simulink model "PassengerCar"  (R2019b)
settings: Solver=ode1  StartTime=0  StopTime=25  FixedStep=1.0000000000000000e-003  RelTol=1e-3
InitFcn:
  | sampleTime = str2double(get_param(bdroot, 'FixedStep'));
undefined symbols (not defined in the file or in its folder): AccPedalPos, BrakePedalPos, BrakeSwitch, DiscIntNeverNeededParam, DYNA4, EngSpd, IgnitionSwitch, InitialGear, InitialSpeed, IntendedEngTrq, LeftIndicator, MainBrakePress, MaxGear, MDL, MinGear, RefAcc, RefLane, RefLatPos, RefPath, RefPathCurv, RefSpd, RefSpdPreview, RefSpdRetrospect, RightIndicator, SteeringWheelAng, SteeringWheelTrq, UserDefinedRefValue, vm_const
libraries: UtilitiesLibrary x31, simulink x18, WheelSystemModules x13, LongitudinalControllerModules x13, LateralControllerModules x7, AnimationBusselectorModules x5, EnvironmentModules x5, BasicEngineControlModules x5, MiscellaneousControlModules x5, Animation3Modules x4, AuxiliariesModules x4, TireModules x4
(part 18 of 39)

== system PassengerCar/Vehicle/Drivetrain/DrivetrainControlUnit/InputFromDrivetrainPhysics ==
  fromDrivetrainPhysics : Inport
  TDBusSelector : BusSelector  OutputSignals=Transmission.Type[-],EngSpd[rad/s],Transmission.InSpd[rad/s],Transmission.OutSpd[rad/s],Transmission.NumFwdGears[-]
  __TDD__EngSpd[rad/s] : Demux  Outputs=[1]
  __TDD__InSpd[rad/s] : Demux  Outputs=[1]
  __TDD__NumFwdGears[-] : Demux  Outputs=[1]
  __TDD__OutSpd[rad/s] : Demux  Outputs=[1]
  __TDD__Type[-] : Demux  Outputs=1
  Type[-]___UNIQUE_1 : Outport  Description=|  VectorParamsAs1DForOutWhenUnconnected=off
      | <name>Transmission.Type[-]</name>
      | <comment></comment>
  EngSpd[rad/s] : Outport  Description=|  Port=2  PortDimensions=[1]  VectorParamsAs1DForOutWhenUnconnected=off
      | <name>EngSpd[rad/s]</name>
      | <comment>Engine speed</comment>
  InSpd[rad/s]___UNIQUE_1 : Outport  Description=|  Port=3  PortDimensions=[1]  VectorParamsAs1DForOutWhenUnconnected=off
      | <name>Transmission.InSpd[rad/s]</name>
      | <comment>Transmission input speed</comment>
  OutSpd[rad/s]___UNIQUE_1 : Outport  Description=|  Port=4  PortDimensions=[1]  VectorParamsAs1DForOutWhenUnconnected=off
      | <name>Transmission.OutSpd[rad/s]</name>
      | <comment>Transmission output speed</comment>
  NumFwdGears[-]___UNIQUE_1 : Outport  Description=|  Port=5  PortDimensions=[1]  VectorParamsAs1DForOutWhenUnconnected=off
      | <name>Transmission.NumFwdGears[-]</name>
      | <comment>Number of forward gears</comment>
  wires:
  __TDD__NumFwdGears[-]/1 -> NumFwdGears[-]___UNIQUE_1/1  "NumFwdGears[-]"
  __TDD__OutSpd[rad/s]/1 -> OutSpd[rad/s]___UNIQUE_1/1  "OutSpd[rad/s]"
  __TDD__InSpd[rad/s]/1 -> InSpd[rad/s]___UNIQUE_1/1  "InSpd[rad/s]"
  __TDD__EngSpd[rad/s]/1 -> EngSpd[rad/s]/1  "EngSpd[rad/s]"
  __TDD__Type[-]/1 -> Type[-]___UNIQUE_1/1  "Type[-]"
  TDBusSelector/5 -> __TDD__NumFwdGears[-]/1  "<NumFwdGears[-]>"
  TDBusSelector/4 -> __TDD__OutSpd[rad/s]/1  "<OutSpd[rad/s]>"
  TDBusSelector/3 -> __TDD__InSpd[rad/s]/1  "<InSpd[rad/s]>"
  TDBusSelector/2 -> __TDD__EngSpd[rad/s]/1  "<EngSpd[rad/s]>"
  TDBusSelector/1 -> __TDD__Type[-]/1  "<Type[-]>"
  fromDrivetrainPhysics/1 -> TDBusSelector/1

== system PassengerCar/Vehicle/Drivetrain/DrivetrainControlUnit/TransmissionControlUnit ==
  AccPedalPos[0_1] : Inport  Description=Accelerator pedal position
  EngSpd[rad/s] : Inport  Description=Engine speed  Port=2
  TransmissionInSpd[rad/s] : Inport  Description=Transmission input speed  Port=3
  TransmissionOutSpd[rad/s] : Inport  Description=Transmission output speed  Port=4
  NumFwdGears[-] : Inport  Description=Number of forward gears  Port=5
  InitialGear[-4;20] : Inport  Description=Accelerator pedal position  Port=6
  MaxGear[-4;20] : Inport  Description=Maximum gear  Port=7
  MinGear[-4;20] : Inport  Description=Minimum gear  Port=8
  ShiftingProgramSelection[-] : Inport  Description=Shifting program selection  Port=9
  KickdownSwitch[0;1] : Inport  Description=Kick-down switch  Port=10
  Enable : EnablePort  StatesWhenEnabling=reset
  TransmissionControlUnit : TransmissionControlModules/TransmissionControlUnit  DATA_NODE=MDL.Vehicle.Drivetrain.DrivetrainControlUnit.TransmissionControlUnit  GearChangeMinTime=MDL.Vehicle.Drivetrain.DrivetrainControlUnit.TransmissionControlUnit.GearChangeMinTime  GearChangeDelay=MDL.Vehicle.Drivetrain.DrivetrainControlUnit.TransmissionControlUnit.GearChangeDelay  EngSpdFilterTimeConst=MDL.Vehicle.Drivetrain.DrivetrainControlUnit.TransmissionControlUnit.EngSpdFilterTimeConst  LockUpClutchOpenTime=MDL.Vehicle.Drivetrain.DrivetrainControlUnit.TransmissionControlUnit.LockUpClutch.OpenTime  LockUpClutchCloseTime=MDL.Vehicle.Drivetrain.DrivetrainControlUnit.TransmissionControlUnit.LockUpClutch.CloseTime  ThresKickdownOpenControlled=MDL.Vehicle.Drivetrain.DrivetrainControlUnit.TransmissionControlUnit.LockUpClutch.KickDownMode.OpenToControlledSpdCurve  ThresKickdownControlledOpen=MDL.Vehicle.Drivetrain.DrivetrainControlUnit.TransmissionControlUnit.LockUpClutch.KickDownMode.ControlledToOpenSpdCurve  ThresKickdownClosedControlled=MDL.Vehicle.Drivetrain.DrivetrainControlUnit.TransmissionControlUnit.LockUpClutch.KickDownMode.ClosedToControlledSpdCurve  ThresKickdownControlledClosed=MDL.Vehicle.Drivetrain.DrivetrainControlUnit.TransmissionControlUnit.LockUpClutch.KickDownMode.ControlledToClosedSpdCurve  ThresOpenControlled=MDL.Vehicle.Drivetrain.DrivetrainControlUnit.TransmissionControlUnit.LockUpClutch.RegularMode.OpenToControlledSpdMap3D  ThresControlledOpen=MDL.Vehicle.Drivetrain.DrivetrainControlUnit.TransmissionControlUnit.LockUpClutch.RegularMode.ControlledToOpenSpdMap3D  ThresClosedControlled=MDL.Vehicle.Drivetrain.DrivetrainControlUnit.TransmissionControlUnit.LockUpClutch.RegularMode.ClosedToControlledSpdMap3D  ThresControlledClosed=MDL.Vehicle.Drivetrain.DrivetrainControlUnit.TransmissionControlUnit.LockUpClutch.RegularMode.ControlledToClosedSpdMap3D  OpenClutchDelay=MDL.Vehicle.Drivetrain.DrivetrainControlUnit.TransmissionControlUnit.ManualClutch.OpenClutchDelay  ClutchPedalCorrectFac=MDL.Vehicle.Drivetrain.DrivetrainControlUnit.TransmissionControlUnit.ManualClutch.ClutchPedalCorrectFacCurve  ClutchOpenTime=MDL.Vehicle.Drivetrain.DrivetrainControlUnit.TransmissionControlUnit.ManualClutch.OpenTime  OpenClutchDuration=MDL.Vehicle.Drivetrain.DrivetrainControlUnit.TransmissionControlUnit.ManualClutch.OpenClutchDuration  ClutchCloseTime=MDL.Vehicle.Drivetrain.DrivetrainControlUnit.TransmissionControlUnit.ManualClutch.CloseTime  LowerGearLimit=MDL.Vehicle.Drivetrain.DrivetrainControlUnit.TransmissionControlUnit.ShiftingProgram.DirectShifting.LowerGearLimit  TransmissionOutSpdThres=MDL.Vehicle.Drivetrain.DrivetrainControlUnit.TransmissionControlUnit.ShiftingProgram.DirectShifting.Spd  KickdownShiftUp=MDL.Vehicle.Drivetrain.DrivetrainControlUnit.TransmissionControlUnit.ShiftingProgram.KickDownMode.UpshiftSpdCurve  KickdownShiftDown=MDL.Vehicle.Drivetrain.DrivetrainControlUnit.TransmissionControlUnit.ShiftingProgram.KickDownMode.DownshiftSpdCurve  ShiftUp=MDL.Vehicle.Drivetrain.DrivetrainControlUnit.TransmissionControlUnit.ShiftingProgram.RegularMode.UpshiftSpdMap3D  ShiftDown=MDL.Vehicle.Drivetrain.DrivetrainControlUnit.TransmissionControlUnit.ShiftingProgram.RegularMode.DownshiftSpdMap3D  SlipCtrlClutchSlip=MDL.Vehicle.Drivetrain.DrivetrainControlUnit.TransmissionControlUnit.SlipController.ClutchIntendedSlipMap3D  SlipCtrlProportionalGain=MDL.Vehicle.Drivetrain.DrivetrainControlUnit.TransmissionControlUnit.SlipController.ProportionalGain  SlipCtrlIntegralGain=MDL.Vehicle.Drivetrain.DrivetrainControlUnit.TransmissionControlUnit.SlipController.IntegralGain  SlipCtrlTimeConst=MDL.Vehicle.Drivetrain.DrivetrainControlUnit.TransmissionControlUnit.SlipController.TimeConst  TractionCtrlIntTrq=MDL.Vehicle.Drivetrain.DrivetrainControlUnit.TransmissionControlUnit.TractionController.RefEngTrq  ASREndClutchPos=MDL.Vehicle.Drivetrain.DrivetrainControlUnit.TransmissionControlUnit.TractionController.ASREndClutchPos
  Gear[-4;20] : Outport  Description=Gear  OutputWhenDisabled=reset  InitialOutput=0  VectorParamsAs1DForOutWhenUnconnected=off
  LockUpClutchPos[0_1] : Outport  Description=Lock-up clutch position  Port=2  OutputWhenDisabled=reset  InitialOutput=0  VectorParamsAs1DForOutWhenUnconnected=off
  AutomatedManualClutchPos[0_1] : Outport  Description=Clutch position for manual shifting  Port=3  OutputWhenDisabled=reset  InitialOutput=0  VectorParamsAs1DForOutWhenUnconnected=off
  GearTarget[-4;20] : Outport  Description=ASR torque  Port=4  OutputWhenDisabled=reset  InitialOutput=0  VectorParamsAs1DForOutWhenUnconnected=off
  ASRRequestSwitch[0;2] : Outport  Description=Switch indicating if no ASR (0), slow ASR (1), or fast ASR (2) is requested  Port=5  OutputWhenDisabled=reset  InitialOutput=0  VectorParamsAs1DForOutWhenUnconnected=off
  ASRTrq[Nm] : Outport  Description=ASR torque  Port=6  OutputWhenDisabled=reset  InitialOutput=0  VectorParamsAs1DForOutWhenUnconnected=off
  wires:
  InitialGear[-4;20]/1 -> TransmissionControlUnit/6
  NumFwdGears[-]/1 -> TransmissionControlUnit/5
  TransmissionOutSpd[rad/s]/1 -> TransmissionControlUnit/4
  EngSpd[rad/s]/1 -> TransmissionControlUnit/2
  AccPedalPos[0_1]/1 -> TransmissionControlUnit/1
  TransmissionInSpd[rad/s]/1 -> TransmissionControlUnit/3
  KickdownSwitch[0;1]/1 -> TransmissionControlUnit/10
  TransmissionControlUnit/6 -> GearTarget[-4;20]/1
  ShiftingProgramSelection[-]/1 -> TransmissionControlUnit/9
  MinGear[-4;20]/1 -> TransmissionControlUnit/8
  MaxGear[-4;20]/1 -> TransmissionControlUnit/7
  TransmissionControlUnit/1 -> Gear[-4;20]/1
  TransmissionControlUnit/2 -> LockUpClutchPos[0_1]/1
  TransmissionControlUnit/3 -> AutomatedManualClutchPos[0_1]/1
  TransmissionControlUnit/4 -> ASRRequestSwitch[0;2]/1
  TransmissionControlUnit/5 -> ASRTrq[Nm]/1

== system PassengerCar/Vehicle/Drivetrain/DrivetrainPhysics/DrivetrainPhysicsInputs ==
  fromEngine : Inport
  fromWheelSystem : Inport  Port=2
  fromCTRL : Inport  Port=3
  fromDrivetrainControlUnit : Inport  Port=4
  fromAuxiliaries : Inport  Port=5
  Add : Sum
  Add1 : Sum
  Add2 : Sum  Inputs=+-
  Bus to Vector : BusToVector
  InputFromAuxiliaries : Subsystem  Tag=TESIS DYNAware Interface Block  mask{NeedsUpdate=off, SignalInfo=|}
      mask SignalInfo=|
      | {
      |   "Version": "4.6",
      |   "MuxedOutputBusName": "output",
      |   "MuxedInputBusName": "fromAuxiliaries",
      |   "MuxedInputSelected": true,
      |   "MuxedOutputSelected": false,
      |   "SignalData": [
      |     {
      |       "initialValue": "0.0",
      |       "name": "StarterInrt[kgm**2]",
      |       "comment": "",
      |       "minString": "",
      |       "maxString": "",
      |       "width": 1,
      |       "dataType": 0,
      |       "signalType": 0,
      |       "createSignal": false,
      |       "outputName": "StarterInrt[kgm**2]",
      |       "generateSignalAccessBlock": false,
      |       "accessId": "$(parentId).$(blockName).$(outputName)"
      |     },
      |     {
      |       "initialValue": "0.0",
      |       "name": "StarterTrq[Nm]",
      |       "comment": "",
      |       "minString": "",
      |       "maxString": "",
      |       "width": 1,
      |       "dataType": 0,
      |       "signalType": 0,
      |       "createSignal": false,
      |       "outputName": "StarterTrq[Nm]",
      |       "generateSignalAccessBlock": false,
      |       "accessId": "$(parentId).$(blockName).$(outputName)"
      |     }
      |   ]
      | }
      mask prompts: NeedsUpdate "Specify, if subsystem content needs to be updated"; SignalInfo "Signal Info (json)"
      mask help: DYNA4 Interface Block Version 4.6
      mask init:
      | blockName = get_param(gcbh, 'Name');
      | parentId = DYNA4.ModelHandling.AccessID.getFromHierarchy(gcbh);
      | TD.InterfaceBlock.ModelCallbacks.GenerateContent(gcb);
      settings: DeleteFcn=TD.InterfaceBlock.ModelCallbacks.CloseGUI( gcbh );  NameChangeFcn=TD.InterfaceBlock.ModelCallbacks.BlockRenamedHandler(gcbh);  OpenFcn=TD.InterfaceBlock.ModelCallbacks.OpenGUI( gcbh );  CloseFcn=TD.InterfaceBlock.ModelCallbacks.CloseGUI( gcbh );
      mask Display:
      | image('InterfaceBlock.png','center');
      | port_label('input',1, 'fromAuxiliaries');
      | port_label('output',1, 'StarterInrt[kgm**2]');
      | port_label('output',2, 'StarterTrq[Nm]');
  InputFromCTRL : Subsystem  Tag=TESIS DYNAware Interface Block  mask{NeedsUpdate=off, SignalInfo=|}
      mask SignalInfo=|
      | {
      |   "Version": "4.6",
      |   "MuxedOutputBusName": "output",
      |   "MuxedInputBusName": "fromCTRL",
      |   "MuxedInputSelected": true,
      |   "MuxedOutputSelected": false,
      |   "SignalData": [
      |     {
      |       "initialValue": "0.0",
      |       "name": "CTRL.LongitudinalControl.InitialEngineSpeed[rad/s]",
      |       "comment": "",
      |       "minString": "",
      |       "maxString": "",
      |       "width": 1,
      |       "dataType": 0,
      |       "signalType": 0,
      |       "createSignal": false,
      |       "outputName": "InitialEngineSpeed[rad/s]",
      |       "generateSignalAccessBlock": false,
      |       "accessId": "$(parentId).$(blockName).$(outputName)"
      |     },
      |     {
      |       "initialValue": "0.0",
      |       "name": "CTRL.LongitudinalControl.InitialGear[-4;20]",
      |       "comment": "",
      |       "minString": "",
      |       "maxString": "",
      |       "width": 1,
      |       "dataType": 0,
      |       "signalType": 0,
      |       "createSignal": false,
      |       "outputName": "InitialGear[-4;20]",
      |       "generateSignalAccessBlock": false,
      |       "accessId": "$(parentId).$(blockName).$(outputName)"
      |     },
      |     {
      |       "initialValue": "0.0",
      |       "name": "CTRL.LongitudinalControl.ClutchPos[0_1]",
      |       "comment": "",
      |       "minString": "",
      |       "maxString": "",
      |       "width": 1,
      |       "dataType": 0,
      |       "signalType": 0,
      |       "createSignal": false,
      |       "outputName": "ClutchPos[0_1]",
      |       "generateSignalAccessBlock": false,
      |       "accessId": "$(parentId).$(blockName).$(outputName)"
      |     },
      |     {
      |       "initialValue": "0.0",
      |       "name": "CTRL.LongitudinalControl.ManualGear[-4;20]",
      |       "comment": "",
      |       "minString": "",
      |       "maxString": "",
      |       "width": 1,
      |       "dataType": 0,
      |       "signalType": 0,
      |       "createSignal": false,
      |       "outputName": "ManualGear[-4;20]",
      |       "generateSignalAccessBlock": false,
      |       "accessId": "$(parentId).$(blockName).$(outputName)"
      |     },
      |     {
      |       "initialValue": "0.0",
      |       "name": "CTRL.LongitudinalControl.TransferCaseLock[0;1]",
      |       "comment": "",
      |       "minString": "",
      |       "maxString": "",
      |       "width": 1,
      |       "dataType": 0,
      |       "signalType": 0,
      |       "createSignal": false,
      |       "outputName": "TransferCaseLock[0;1]",
      |       "generateSignalAccessBlock": false,
      |       "accessId": "$(parentId).$(blockName).$(outputName)"
      |     },
      |     {
      |       "initialValue": "0.0",
      |       "name": "CTRL.LongitudinalControl.FrontDifferentialLock[0;1]",
      |       "comment": "",
      |       "minString": "",
      |       "maxString": "",
      |       "width": 1,
      |       "dataType": 0,
      |       "signalType": 0,
      |       "createSignal": false,
      |       "outputName": "FrontDifferentialLock[0;1]",
      |       "generateSignalAccessBlock": false,
      |       "accessId": "$(parentId).$(blockName).$(outputName)"
      |     },
      |     {
      |       "initialValue": "0.0",
      |       "name": "CTRL.LongitudinalControl.RearDifferentialLock[0;1]",
      |       "comment": "",
      |       "minString": "",
      |       "maxString": "",
      |       "width": 1,
      |       "dataType": 0,
      |       "signalType": 0,
      |       "createSignal": false,
      |       "outputName": "RearDifferentialLock[0;1]",
      |       "generateSignalAccessBlock": false,
      |       "accessId": "$(parentId).$(blockName).$(outputName)"
      |     },
      |     {
      |       "initialValue": "0.0",
      |       "name": "CTRL.LongitudinalControl.Rear2DifferentialLock[0;1]",
      |       "comment": "",
      |       "minString": "",
      |       "maxString": "",
      |       "width": 1,
      |       "dataType": 0,
      |       "signalType": 0,
      |       "createSignal": false,
      |       "outputName": "Rear2DifferentialLock[0;1]",
      |       "generateSignalAccessBlock": false,
      |       "accessId": "$(parentId).$(blockName).$(outputName)"
      |     },
      |     {
      |       "initialValue": "0.0",
      |       "name": "CTRL.LongitudinalControl.Rear3DifferentialLock[0;1]",
      |       "comment": "",
      |       "minString": "",
      |       "maxString": "",
      |       "width": 1,
      |       "dataType": 0,
      |       "signalType": 0,
      |       "createSignal": false,
      |       "outputName": "Rear3DifferentialLock[0;1]",
      |       "generateSignalAccessBlock": false,
      |       "accessId": "$(parentId).$(blockName).$(outputName)"
      |     },
      |     {
      |       "initialValue": "0.0",
      |       "name": "CTRL.TemperatureControl.TransmissionTemp[K]",
      |       "comment": "",
      |       "minString": "",
      |       "maxString": "",
      |       "width": 1,
      |       "dataType": 0,
      |       "signalType": 0,
      |       "createSignal": false,
      |       "outputName": "TransmissionTemp[K]",
      |       "generateSignalAccessBlock": false,
      |       "accessId": "$(parentId).$(blockName).$(outputName)"
      |     },
      |     {
      |       "initialValue": "0.0",
      |       "name": "CTRL.TemperatureControl.TransferCaseTemp[K]",
      |       "comment": "",
      |       "minString": "",
      |       "maxString": "",
      |       "width": 1,
      |       "dataType": 0,
      |       "signalType": 0,
      |       "createSignal": false,
      |       "outputName": "TransferCaseTemp[K]",
      |       "generateSignalAccessBlock": false,
      |       "accessId": "$(parentId).$(blockName).$(outputName)"
      |     },
      |     {
      |       "initialValue": "0.0",
      |       "name": "CTRL.TemperatureControl.FrontDifferentialTemp[K]",
      |       "comment": "",
      |       "minString": "",
      |       "maxString": "",
      |       "width": 1,
      |       "dataType": 0,
      |       "signalType": 0,
      |       "createSignal": false,
      |       "outputName": "FrontDifferentialTemp[K]",
      |       "generateSignalAccessBlock": false,
      |       "accessId": "$(parentId).$(blockName).$(outputName)"
      |     },
      |     {
      |       "initialValue": "0.0",
      |       "name": "CTRL.TemperatureControl.RearDifferentialTemp[K]",
      |       "comment": "",
      |       "minString": "",
      |       "maxString": "",
      |       "width": 1,
      |       "dataType": 0,
      |       "signalType": 0,
      |       "createSignal": false,
      |       "outputName": "RearDifferentialTemp[K]",
      |       "generateSignalAccessBlock": false,
      |       "accessId": "$(parentId).$(blockName).$(outputName)"
      |     },
      |     {
      |       "initialValue": "0.0",
      |       "name": "CTRL.TemperatureControl.Rear2DifferentialTemp[K]",
      |       "comment": "",
      |       "minString": "",
      |       "maxString": "",
      |       "width": 1,
      |       "dataType": 0,
      |       "signalType": 0,
      |       "createSignal": false,
      |       "outputName": "Rear2DifferentialTemp[K]",
      |       "generateSignalAccessBlock": false,
      |       "accessId": "$(parentId).$(blockName).$(outputName)"
      |     },
      |     {
      |       "initialValue": "0.0",
      |       "name": "CTRL.TemperatureControl.Rear3DifferentialTemp[K]",
      |       "comment": "",
      |       "minString": "",
      |       "maxString": "",
      |       "width": 1,
      |       "dataType": 0,
      |       "signalType": 0,
      |       "createSignal": false,
      |       "outputName": "Rear3DifferentialTemp[K]",
      |       "generateSignalAccessBlock": false,
      |       "accessId": "$(parentId).$(blockName).$(outputName)"
      |     }
      |   ]
      | }
      mask prompts: NeedsUpdate "Specify, if subsystem content needs to be updated"; SignalInfo "Signal Info (json)"
      mask help: DYNA4 Interface Block Version 4.6
      mask init:
      | blockName = get_param(gcbh, 'Name');
      | parentId = DYNA4.ModelHandling.AccessID.getFromHierarchy(gcbh);
      | TD.InterfaceBlock.ModelCallbacks.GenerateContent(gcb);
      settings: DeleteFcn=TD.InterfaceBlock.ModelCallbacks.CloseGUI( gcbh );  NameChangeFcn=TD.InterfaceBlock.ModelCallbacks.BlockRenamedHandler(gcbh);  OpenFcn=TD.InterfaceBlock.ModelCallbacks.OpenGUI( gcbh );  CloseFcn=TD.InterfaceBlock.ModelCallbacks.CloseGUI( gcbh );
      mask Display:
      | image('InterfaceBlock.png','center');
      | port_label('input',1, 'fromCTRL');
      | port_label('output',1, 'InitialEngineSpeed[rad/s]');
      | port_label('output',2, 'InitialGear[-4;20]');
      | port_label('output',3, 'ClutchPos[0_1]');
      | port_label('output',4, 'ManualGear[-4;20]');
      | port_label('output',5, 'TransferCaseLock[0;1]');
      | port_label('output',6, 'FrontDifferentialLock[0;1]');
      | port_label('output',7, 'RearDifferentialLock[0;1]');
      | port_label('output',8, 'Rear2DifferentialLock[0;1]');
      | port_label('output',9, 'Rear3DifferentialLock[0;1]');
      | port_label('output',10, 'TransmissionTemp[K]');
      | port_label('output',11, 'TransferCaseTemp[K]');
      | port_label('output',12, 'FrontDifferentialTemp[K]');
      | port_label('output',13, 'RearDifferentialTemp[K]');
      | port_label('output',14, 'Rear2DifferentialTemp[K]');
      | port_label('output',15, 'Rear3DifferentialTemp[K]');
  InputFromDrivetrainControlUnit : Subsystem  Tag=TESIS DYNAware Interface Block  mask{NeedsUpdate=off, SignalInfo=|}
      mask SignalInfo=|
      | {
      |   "Version": "4.6",
      |   "MuxedOutputBusName": "output",
      |   "MuxedInputBusName": "fromDrivetrainControlUnit",
      |   "MuxedInputSelected": true,
      |   "MuxedOutputSelected": false,
      |   "SignalData": [
      |     {
      |       "initialValue": "0.0",
      |       "name": "TransmissionControlUnit.AutomatedManualClutchPos[0_1]",
      |       "comment": "",
      |       "minString": "",
      |       "maxString": "",
      |       "width": 1,
      |       "dataType": 0,
      |       "signalType": 0,
      |       "createSignal": false,
      |       "outputName": "AutomatedManualClutchPos[0_1]",
      |       "generateSignalAccessBlock": false,
      |       "accessId": "$(parentId).$(blockName).$(outputName)"
      |     },
      |     {
      |       "initialValue": "0.0",
      |       "name": "TransmissionControlUnit.LockUpClutchPos[0_1]",
      |       "comment": "",
      |       "minString": "",
      |       "maxString": "",
      |       "width": 1,
      |       "dataType": 0,
      |       "signalType": 0,
      |       "createSignal": false,
      |       "outputName": "LockUpClutchPos[0_1]",
      |       "generateSignalAccessBlock": false,
      |       "accessId": "$(parentId).$(blockName).$(outputName)"
      |     },
      |     {
      |       "initialValue": "0.0",
      |       "name": "TransmissionControlUnit.Gear[-4;20]",
      |       "comment": "",
      |       "minString": "",
      |       "maxString": "",
      |       "width": 1,
      |       "dataType": 0,
      |       "signalType": 0,
      |       "createSignal": false,
      |       "outputName": "AutomaticGear[-4;20]",
      |       "generateSignalAccessBlock": false,
      |       "accessId": "$(parentId).$(blockName).$(outputName)"
      |     }
      |   ]
      | }
      mask prompts: NeedsUpdate "Specify, if subsystem content needs to be updated"; SignalInfo "Signal Info (json)"
      mask help: DYNA4 Interface Block Version 4.6
      mask init:
      | blockName = get_param(gcbh, 'Name');
      | parentId = DYNA4.ModelHandling.AccessID.getFromHierarchy(gcbh);
      | TD.InterfaceBlock.ModelCallbacks.GenerateContent(gcb);
      settings: DeleteFcn=TD.InterfaceBlock.ModelCallbacks.CloseGUI( gcbh );  NameChangeFcn=TD.InterfaceBlock.ModelCallbacks.BlockRenamedHandler(gcbh);  OpenFcn=TD.InterfaceBlock.ModelCallbacks.OpenGUI( gcbh );  CloseFcn=TD.InterfaceBlock.ModelCallbacks.CloseGUI( gcbh );
      mask Display:
      | image('InterfaceBlock.png','center');
      | port_label('input',1, 'fromDrivetrainControlUnit');
      | port_label('output',1, 'AutomatedManualClutchPos[0_1]');
      | port_label('output',2, 'LockUpClutchPos[0_1]');
      | port_label('output',3, 'AutomaticGear[-4;20]');
  InputFromEngine : Subsystem  Tag=TESIS DYNAware Interface Block  mask{NeedsUpdate=off, SignalInfo=|}
      mask SignalInfo=|
      | {
      |   "Version": "4.6",
      |   "MuxedOutputBusName": "Drivetrain",
      |   "MuxedInputBusName": "fromEngine",
      |   "MuxedInputSelected": true,
      |   "MuxedOutputSelected": false,
      |   "SignalData": [
      |     {
      |       "initialValue": "0.0",
      |       "name": "EnginePhysics.Mechanics.EngInrt[kg*m**2]",
      |       "comment": "",
      |       "minString": "",
      |       "maxString": "",
      |       "width": 1,
      |       "dataType": 0,
      |       "signalType": 0,
      |       "createSignal": false,
      |       "outputName": "EngInrt[kg*m**2]",
      |       "generateSignalAccessBlock": false,
      |       "accessId": "$(parentId).$(blockName).$(outputName)"
      |     },
      |     {
      |       "initialValue": "0.0",
      |       "name": "EnginePhysics.Mechanics.EngTrq[Nm]",
      |       "comment": "",
      |       "minString": "",
      |       "maxString": "",
      |       "width": 1,
      |       "dataType": 0,
      |       "signalType": 0,
      |       "createSignal": false,
      |       "outputName": "EngTrq[Nm]",
      |       "generateSignalAccessBlock": false,
      |       "accessId": "$(parentId).$(blockName).$(outputName)"
      |     },
      |     {
      |       "initialValue": "0.0",
      |       "name": "EnginePhysics.Mechanics.DerivativeOfEngTrq_wrt_CrankAng[Nm/rad]",
      |       "comment": "",
      |       "minString": "",
      |       "maxString": "",
      |       "width": 1,
      |       "dataType": 0,
      |       "signalType": 0,
      |       "createSignal": false,
      |       "outputName": "DerivativeOfEngTrq_wrt_CrankAng[Nm/rad]",
      |       "generateSignalAccessBlock": false,
      |       "accessId": "$(parentId).$(blockName).$(outputName)"
      |     },
      |     {
      |       "initialValue": "0.0",
      |       "name": "EnginePhysics.Mechanics.DerivativeOfEngTrq_wrt_EngSpd[Nm/(rad/s)]",
      |       "comment": "",
      |       "minString": "",
      |       "maxString": "",
      |       "width": 1,
      |       "dataType": 0,
      |       "signalType": 0,
      |       "createSignal": false,
      |       "outputName": "DerivativeOfEngTrq_wrt_EngSpd[Nm/(rad/s)]",
      |       "generateSignalAccessBlock": false,
      |       "accessId": "$(parentId).$(blockName).$(outputName)"
      |     },
      |     {
      |       "initialValue": "0.0",
      |       "name": "EnginePhysics.Mechanics.MeanEngFrictionTrq[Nm]",
      |       "comment": "",
      |       "minString": "",
      |       "maxString": "",
      |       "width": 1,
      |       "dataType": 0,
      |       "signalType": 0,
      |       "createSignal": false,
      |       "outputName": "MeanEngFrictionTrq[Nm]",
      |       "generateSignalAccessBlock": false,
      |       "accessId": "$(parentId).$(blockName).$(outputName)"
      |     },
      |     {
      |       "initialValue": "0.0",
      |       "name": "EngineControlUnit.EngIdleSpd[rad/s]",
      |       "comment": "",
      |       "minString": "",
      |       "maxString": "",
      |       "width": 1,
      |       "dataType": 0,
      |       "signalType": 0,
      |       "createSignal": false,
      |       "outputName": "EngIdleSpd[rad/s]",
      |       "generateSignalAccessBlock": false,
      |       "accessId": "$(parentId).$(blockName).$(outputName)"
      |     }
      |   ]
      | }
      mask prompts: NeedsUpdate "Specify, if subsystem content needs to be updated"; SignalInfo "Signal Info (json)"
      mask help: DYNA4 Interface Block Version 4.6
      mask init:
      | blockName = get_param(gcbh, 'Name');
      | parentId = DYNA4.ModelHandling.AccessID.getFromHierarchy(gcbh);
      | TD.InterfaceBlock.ModelCallbacks.GenerateContent(gcb);
      settings: DeleteFcn=TD.InterfaceBlock.ModelCallbacks.CloseGUI( gcbh );  NameChangeFcn=TD.InterfaceBlock.ModelCallbacks.BlockRenamedHandler(gcbh);  OpenFcn=TD.InterfaceBlock.ModelCallbacks.OpenGUI( gcbh );  CloseFcn=TD.InterfaceBlock.ModelCallbacks.CloseGUI( gcbh );
      mask Display:
      | image('InterfaceBlock.png','center');
      | port_label('input',1, 'fromEngine');
      | port_label('output',1, 'EngInrt[kg*m**2]');
      | port_label('output',2, 'EngTrq[Nm]');
      | port_label('output',3, 'DerivativeOfEngTrq_wrt_CrankAng[Nm/rad]');
      | port_label('output',4, 'DerivativeOfEngTrq_wrt_EngSpd[Nm/(rad/s)]');
      | port_label('output',5, 'MeanEngFrictionTrq[Nm]');
      | port_label('output',6, 'EngIdleSpd[rad/s]');
  InputFromWheelSystem : Subsystem  Tag=TESIS DYNAware Interface Block  mask{NeedsUpdate=off, SignalInfo=|}
      mask SignalInfo=|
      | {
      |   "Version": "4.6",
      |   "MuxedOutputBusName": "WheelSystem",
      |   "MuxedInputBusName": "fromWheelSystem",
      |   "MuxedInputSelected": true,
      |   "MuxedOutputSelected": true,
      |   "SignalData": [
      |     {
      |       "initialValue": "0.0",
      |       "name": "FrontLeft.Wheel.RotSpd[rad/s]",
      |       "comment": "",
      |       "minString": "",
      |       "maxString": "",
      |       "width": 1,
      |       "dataType": 0,
      |       "signalType": 0,
      |       "createSignal": false,
      |       "outputName": "RotSpdFL[rad/s]",
      |       "generateSignalAccessBlock": false,
      |       "accessId": "$(parentId).$(blockName).$(outputName)"
      |     },
      |     {
      |       "initialValue": "0.0",
      |       "name": "FrontRight.Wheel.RotSpd[rad/s]",
      |       "comment": "",
      |       "minString": "",
      |       "maxString": "",
      |       "width": 1,
      |       "dataType": 0,
      |       "signalType": 0,
      |       "createSignal": false,
      |       "outputName": "RotSpdFR[rad/s]",
      |       "generateSignalAccessBlock": false,
      |       "accessId": "$(parentId).$(blockName).$(outputName)"
      |     },
      |     {
      |       "initialValue": "0.0",
      |       "name": "RearLeft.Wheel.RotSpd[rad/s]",
      |       "comment": "",
      |       "minString": "",
      |       "maxString": "",
      |       "width": 1,
      |       "dataType": 0,
      |       "signalType": 0,
      |       "createSignal": false,
      |       "outputName": "RotSpdRL[rad/s]",
      |       "generateSignalAccessBlock": false,
      |       "accessId": "$(parentId).$(blockName).$(outputName)"
      |     },
      |     {
      |       "initialValue": "0.0",
      |       "name": "RearRight.Wheel.RotSpd[rad/s]",
      |       "comment": "",
      |       "minString": "",
      |       "maxString": "",
      |       "width": 1,
      |       "dataType": 0,
      |       "signalType": 0,
      |       "createSignal": false,
      |       "outputName": "RotSpdRR[rad/s]",
      |       "generateSignalAccessBlock": false,
      |       "accessId": "$(parentId).$(blockName).$(outputName)"
      |     },
      |     {
      |       "initialValue": "0.0",
      |       "name": "Rear2Left.Wheel.RotSpd[rad/s]",
      |       "comment": "",
      |       "minString": "",
      |       "maxString": "",
      |       "width": 1,
      |       "dataType": 0,
      |       "signalType": 0,
      |       "createSignal": false,
      |       "outputName": "RotSpdR2L[rad/s]",
      |       "generateSignalAccessBlock": false,
      |       "accessId": "$(parentId).$(blockName).$(outputName)"
      |     },
      |     {
      |       "initialValue": "0.0",
      |       "name": "Rear2Right.Wheel.RotSpd[rad/s]",
      |       "comment": "",
      |       "minString": "",
      |       "maxString": "",
      |       "width": 1,
      |       "dataType": 0,
      |       "signalType": 0,
      |       "createSignal": false,
      |       "outputName": "RotSpdR2R[rad/s]",
      |       "generateSignalAccessBlock": false,
      |       "accessId": "$(parentId).$(blockName).$(outputName)"
      |     },
      |     {
      |       "initialValue": "0.0",
      |       "name": "Rear3Left.Wheel.RotSpd[rad/s]",
      |       "comment": "",
      |       "minString": "",
      |       "maxString": "",
      |       "width": 1,
      |       "dataType": 0,
      |       "signalType": 0,
      |       "createSignal": false,
      |       "outputName": "RotSpdR3L[rad/s]",
      |       "generateSignalAccessBlock": false,
      |       "accessId": "$(parentId).$(blockName).$(outputName)"
      |     },
      |     {
      |       "initialValue": "0.0",
      |       "name": "Rear3Right.Wheel.RotSpd[rad/s]",
      |       "comment": "",
      |       "minString": "",
      |       "maxString": "",
      |       "width": 1,
      |       "dataType": 0,
      |       "signalType": 0,
      |       "createSignal": false,
      |       "outputName": "RotSpdR3R[rad/s]",
      |       "generateSignalAccessBlock": false,
      |       "accessId": "$(parentId).$(blockName).$(outputName)"
      |     }
      |   ]
      | }
      mask prompts: NeedsUpdate "Specify, if subsystem content needs to be updated"; SignalInfo "Signal Info (json)"
      mask help: DYNA4 Interface Block Version 4.6
      mask init:
      | blockName = get_param(gcbh, 'Name');
      | parentId = DYNA4.ModelHandling.AccessID.getFromHierarchy(gcbh);
      | TD.InterfaceBlock.ModelCallbacks.GenerateContent(gcb);
      settings: DeleteFcn=TD.InterfaceBlock.ModelCallbacks.CloseGUI( gcbh );  NameChangeFcn=TD.InterfaceBlock.ModelCallbacks.BlockRenamedHandler(gcbh);  OpenFcn=TD.InterfaceBlock.ModelCallbacks.OpenGUI( gcbh );  CloseFcn=TD.InterfaceBlock.ModelCallbacks.CloseGUI( gcbh );
      mask Display:
      | image('InterfaceBlock.png','center');
      | port_label('input',1, 'fromWheelSystem');
      | port_label('output',1, 'WheelSystem');
  Memory1 : Memory  InheritSampleTime=on
  Memory2 : Memory  InheritSampleTime=on
  Memory4 : Memory  InheritSampleTime=on
  Mux1 : Mux  Inputs=16
  Mux2 : Mux  Inputs=[1 1 1 1 1]
  Use IdleSpd if InitialEngineSpeed < 0 : Switch
  InitEngSpd[rad/s] : Outport  VectorParamsAs1DForOutWhenUnconnected=off
  InitialGear[-4;20] : Outport  Port=2  VectorParamsAs1DForOutWhenUnconnected=off
  FromEngine : Outport  Port=3  VectorParamsAs1DForOutWhenUnconnected=off
  FromCTRL : Outport  Port=4  VectorParamsAs1DForOutWhenUnconnected=off
  FromWheelSystem : Outport  Port=5  VectorParamsAs1DForOutWhenUnconnected=off
  wires:
  InputFromCTRL/3(ClutchPos[0_1]___UNIQUE_1) -> Mux1/1
  InputFromCTRL/4(ManualGear[-4;20]___UNIQUE_1) -> Mux1/4
  InputFromCTRL/1(InitialEngineSpeed[rad/s]___UNIQUE_1) -> Use IdleSpd if InitialEngineSpeed < 0/1, Use IdleSpd if InitialEngineSpeed < 0/2
  Use IdleSpd if InitialEngineSpeed < 0/1 -> InitEngSpd[rad/s]/1
  Mux1/1 -> FromCTRL/1
  InputFromCTRL/2(InitialGear[-4;20]___UNIQUE_1) -> InitialGear[-4;20]/1
  Bus to Vector/1 -> FromWheelSystem/1
  fromWheelSystem/1 -> InputFromWheelSystem/1(fromWheelSystem)
  InputFromWheelSystem/1(WheelSystem___UNIQUE_1) -> Bus to Vector/1
  fromCTRL/1 -> InputFromCTRL/1(fromCTRL)
  fromAuxiliaries/1 -> InputFromAuxiliaries/1(fromAuxiliaries)
  fromEngine/1 -> InputFromEngine/1(fromEngine)
  Mux2/1 -> FromEngine/1
  InputFromEngine/3(DerivativeOfEngTrq_wrt_CrankAng[Nm/rad]___UNIQUE_1) -> Mux2/3
  InputFromEngine/4(DerivativeOfEngTrq_wrt_EngSpd[Nm/(rad/s)]___UNIQUE_1) -> Mux2/4
  Add/1 -> Mux2/1
  Add1/1 -> Mux2/2
  InputFromEngine/5(MeanEngFrictionTrq[Nm]___UNIQUE_1) -> Mux2/5, Add2/2
  InputFromAuxiliaries/2(StarterTrq[Nm]___UNIQUE_1) -> Add1/2
  InputFromEngine/2(EngTrq[Nm]___UNIQUE_1) -> Add2/1
  Add2/1 -> Add1/1
  InputFromEngine/1(EngInrt[kg*m**2]___UNIQUE_1) -> Add/1
  InputFromAuxiliaries/1(StarterInrt[kgm**2]___UNIQUE_1) -> Add/2
  Memory4/1 -> Mux1/2
  Memory1/1 -> Mux1/3
  Memory2/1 -> Mux1/5
  InputFromCTRL/5(TransferCaseLock[0;1]___UNIQUE_1) -> Mux1/6
  InputFromCTRL/6(FrontDifferentialLock[0;1]___UNIQUE_1) -> Mux1/7
  InputFromCTRL/7(RearDifferentialLock[0;1]___UNIQUE_1) -> Mux1/8
  InputFromCTRL/8(Rear2DifferentialLock[0;1]___UNIQUE_1) -> Mux1/9
  InputFromCTRL/9(Rear3DifferentialLock[0;1]___UNIQUE_1) -> Mux1/10
  InputFromCTRL/10(TransmissionTemp[K]___UNIQUE_1) -> Mux1/11
  InputFromCTRL/11(TransferCaseTemp[K]___UNIQUE_1) -> Mux1/12
  InputFromCTRL/12(FrontDifferentialTemp[K]___UNIQUE_1) -> Mux1/13
  InputFromCTRL/13(RearDifferentialTemp[K]___UNIQUE_1) -> Mux1/14
  InputFromCTRL/14(Rear2DifferentialTemp[K]___UNIQUE_1) -> Mux1/15
  InputFromCTRL/15(Rear3DifferentialTemp[K]___UNIQUE_1) -> Mux1/16
  fromDrivetrainControlUnit/1 -> InputFromDrivetrainControlUnit/1(fromDrivetrainControlUnit)
  InputFromEngine/6(EngIdleSpd[rad/s]___UNIQUE_1) -> Use IdleSpd if InitialEngineSpeed < 0/3
  InputFromDrivetrainControlUnit/1(AutomatedManualClutchPos[0_1]___UNIQUE_1) -> Memory4/1
  InputFromDrivetrainControlUnit/2(LockUpClutchPos[0_1]___UNIQUE_1) -> Memory1/1
  InputFromDrivetrainControlUnit/3(AutomaticGear[-4;20]___UNIQUE_1) -> Memory2/1

== system PassengerCar/Vehicle/Drivetrain/DrivetrainPhysics/DrivetrainPhysicsOutputs ==
  EngStates : Inport
  ShaftStates : Inport  Port=2
  DrivetrainStates : Inport  Port=3
  ClutchOutput : Subsystem
  Demux : Demux  Outputs=[10 10 10 10]
  Demux{1..3,6} (4 alike) : Demux  Outputs=[5 5]
  Demux5 : Demux  Outputs=[1 1]
  Demux7 : Demux  Outputs=[2 2+6 5 2]
  Demux8 : Demux  Outputs=[1 1 1 1 1]
  DrivetrainPhysicsOutput : Subsystem  Tag=TESIS DYNAware Interface Block  mask{NeedsUpdate=off, SignalInfo=|}
      mask SignalInfo=|
      | {
      |   "Version": "4.6",
      |   "MuxedOutputBusName": "DrivetrainPhysics",
      |   "MuxedInputBusName": "input",
      |   "MuxedInputSelected": false,
      |   "MuxedOutputSelected": true,
      |   "SignalData": [
      |     {
      |       "initialValue": "0.0",
      |       "name": "EngSpd[rad/s]",
      |       "comment": "",
      |       "minString": "",
      |       "maxString": "",
      |       "width": 1,
      |       "dataType": 0,
      |       "signalType": 0,
      |       "createSignal": false,
      |       "outputName": "EngSpd[rad/s]",
      |       "generateSignalAccessBlock": false,
      |       "accessId": "$(parentId).$(blockName).$(outputName)"
      |     },
      |     {
      |       "initialValue": "0.0",
      |       "name": "EngAcc[rad/s**2]",
      |       "comment": "",
      |       "minString": "",
      |       "maxString": "",
      |       "width": 1,
      |       "dataType": 0,
      |       "signalType": 0,
      |       "createSignal": false,
      |       "outputName": "EngAcc[rad/s**2]",
      |       "generateSignalAccessBlock": false,
      |       "accessId": "$(parentId).$(blockName).$(outputName)"
      |     },
      |     {
      |       "initialValue": "0.0",
      |       "name": "Clutch",
      |       "comment": "",
      |       "minString": "",
      |       "maxString": "",
      |       "width": -1,
      |       "dataType": 0,
      |       "signalType": 1,
      |       "createSignal": false,
      |       "outputName": "Clutch",
      |       "generateSignalAccessBlock": false,
      |       "accessId": "$(parentId).$(blockName).$(outputName)"
      |     },
      |     {
      |       "initialValue": "0.0",
      |       "name": "Transmission",
      |       "comment": "",
      |       "minString": "",
      |       "maxString": "",
      |       "width": -1,
      |       "dataType": 0,
      |       "signalType": 1,
      |       "createSignal": false,
      |       "outputName": "Transmission",
      |       "generateSignalAccessBlock": false,
      |       "accessId": "$(parentId).$(blockName).$(outputName)"
      |     },
      |     {
      |       "initialValue": "0.0",
      |       "name": "TransferCase",
      |       "comment": "",
      |       "minString": "",
      |       "maxString": "",
      |       "width": -1,
      |       "dataType": 0,
      |       "signalType": 1,
      |       "createSignal": false,
      |       "outputName": "TransferCase",
      |       "generateSignalAccessBlock": false,
      |       "accessId": "$(parentId).$(blockName).$(outputName)"
      |     },
      |     {
      |       "initialValue": "0.0",
      |       "name": "FrontDifferential",
      |       "comment": "",
      |       "minString": "",
      |       "maxString": "",
      |       "width": -1,
      |       "dataType": 0,
      |       "signalType": 1,
      |       "createSignal": false,
      |       "outputName": "FrontDifferential",
      |       "generateSignalAccessBlock": false,
      |       "accessId": "$(parentId).$(blockName).$(outputName)"
      |     },
      |     {
      |       "initialValue": "0.0",
      |       "name": "FrontLeftShaft",
      |       "comment": "",
      |       "minString": "",
      |       "maxString": "",
      |       "width": -1,
      |       "dataType": 0,
      |       "signalType": 1,
      |       "createSignal": false,
      |       "outputName": "FrontLeftShaft",
      |       "generateSignalAccessBlock": false,
      |       "accessId": "$(parentId).$(blockName).$(outputName)"
      |     },
      |     {
      |       "initialValue": "0.0",
      |       "name": "FrontRightShaft",
      |       "comment": "",
      |       "minString": "",
      |       "maxString": "",
      |       "width": -1,
      |       "dataType": 0,
      |       "signalType": 1,
      |       "createSignal": false,
      |       "outputName": "FrontRightShaft",
      |       "generateSignalAccessBlock": false,
      |       "accessId": "$(parentId).$(blockName).$(outputName)"
      |     },
      |     {
      |       "initialValue": "0.0",
      |       "name": "RearDifferential",
      |       "comment": "",
      |       "minString": "",
      |       "maxString": "",
      |       "width": -1,
      |       "dataType": 0,
      |       "signalType": 1,
      |       "createSignal": false,
      |       "outputName": "RearDifferential",
      |       "generateSignalAccessBlock": false,
      |       "accessId": "$(parentId).$(blockName).$(outputName)"
      |     },
      |     {
      |       "initialValue": "0.0",
      |       "name": "RearLeftShaft",
      |       "comment": "",
      |       "minString": "",
      |       "maxString": "",
      |       "width": -1,
      |       "dataType": 0,
      |       "signalType": 1,
      |       "createSignal": false,
      |       "outputName": "RearLeftShaft",
      |       "generateSignalAccessBlock": false,
      |       "accessId": "$(parentId).$(blockName).$(outputName)"
      |     },
      |     {
      |       "initialValue": "0.0",
      |       "name": "RearRightShaft",
      |       "comment": "",
      |       "minString": "",
      |       "maxString": "",
      |       "width": -1,
      |       "dataType": 0,
      |       "signalType": 1,
      |       "createSignal": false,
      |       "outputName": "RearRightShaft",
      |       "generateSignalAccessBlock": false,
      |       "accessId": "$(parentId).$(blockName).$(outputName)"
      |     },
      |     {
      |       "initialValue": "0.0",
      |       "name": "Rear2Differential",
      |       "comment": "",
      |       "minString": "",
      |       "maxString": "",
      |       "width": -1,
      |       "dataType": 0,
      |       "signalType": 1,
      |       "createSignal": false,
      |       "outputName": "Rear2Differential",
      |       "generateSignalAccessBlock": false,
      |       "accessId": "$(parentId).$(blockName).$(outputName)"
      |     },
      |     {
      |       "initialValue": "0.0",
      |       "name": "Rear2LeftShaft",
      |       "comment": "",
      |       "minString": "",
      |       "maxString": "",
      |       "width": -1,
      |       "dataType": 0,
      |       "signalType": 1,
      |       "createSignal": false,
      |       "outputName": "Rear2LeftShaft",
      |       "generateSignalAccessBlock": false,
      |       "accessId": "$(parentId).$(blockName).$(outputName)"
      |     },
      |     {
      |       "initialValue": "0.0",
      |       "name": "Rear2RightShaft",
      |       "comment": "",
      |       "minString": "",
      |       "maxString": "",
      |       "width": -1,
      |       "dataType": 0,
      |       "signalType": 1,
      |       "createSignal": false,
      |       "outputName": "Rear2RightShaft",
      |       "generateSignalAccessBlock": false,
      |       "accessId": "$(parentId).$(blockName).$(outputName)"
      |     },
      |     {
      |       "initialValue": "0.0",
      |       "name": "Rear3Differential",
      |       "comment": "",
      |       "minString": "",
      |       "maxString": "",
      |       "width": -1,
      |       "dataType": 0,
      |       "signalType": 1,
      |       "createSignal": false,
      |       "outputName": "Rear3Differential",
      |       "generateSignalAccessBlock": false,
      |       "accessId": "$(parentId).$(blockName).$(outputName)"
      |     },
      |     {
      |       "initialValue": "0.0",
      |       "name": "Rear3LeftShaft",
      |       "comment": "",
      |       "minString": "",
      |       "maxString": "",
      |       "width": -1,
      |       "dataType": 0,
      |       "signalType": 1,
      |       "createSignal": false,
      |       "outputName": "Rear3LeftShaft",
      |       "generateSignalAccessBlock": false,
      |       "accessId": "$(parentId).$(blockName).$(outputName)"
      |     },
      |     {
      |       "initialValue": "0.0",
      |       "name": "Rear3RightShaft",
      |       "comment": "",
      |       "minString": "",
      |       "maxString": "",
      |       "width": -1,
      |       "dataType": 0,
      |       "signalType": 1,
      |       "createSignal": false,
      |       "outputName": "Rear3RightShaft",
      |       "generateSignalAccessBlock": false,
      |       "accessId": "$(parentId).$(blockName).$(outputName)"
      |     },
      |     {
      |       "initialValue": "0.0",
      |       "name": "TotalRatio[-]",
      |       "comment": "",
      |       "minString": "",
      |       "maxString": "",
      |       "width": 1,
      |       "dataType": 0,
      |       "signalType": 0,
      |       "createSignal": false,
      |       "outputName": "TotalRatio[-]",
      |       "generateSignalAccessBlock": false,
      |       "accessId": "$(parentId).$(blockName).$(outputName)"
      |     }
      |   ]
      | }
      mask prompts: NeedsUpdate "Specify, if subsystem content needs to be updated"; SignalInfo "Signal Info (json)"
      mask help: DYNA4 Interface Block Version 4.6
      mask init:
      | blockName = get_param(gcbh, 'Name');
      | parentId = DYNA4.ModelHandling.AccessID.getFromHierarchy(gcbh);
      | TD.InterfaceBlock.ModelCallbacks.GenerateContent(gcb);
      settings: DeleteFcn=TD.InterfaceBlock.ModelCallbacks.CloseGUI( gcbh );  NameChangeFcn=TD.InterfaceBlock.ModelCallbacks.BlockRenamedHandler(gcbh);  OpenFcn=TD.InterfaceBlock.ModelCallbacks.OpenGUI( gcbh );  CloseFcn=TD.InterfaceBlock.ModelCallbacks.CloseGUI( gcbh );
      mask Display:
      | image('InterfaceBlock.png','center');
      | port_label('input',1, 'EngSpd[rad/s]');
      | port_label('input',2, 'EngAcc[rad/s**2]');
      | port_label('input',3, 'Clutch');
      | port_label('input',4, 'Transmission');
      | port_label('input',5, 'TransferCase');
      | port_label('input',6, 'FrontDifferential');
      | port_label('input',7, 'FrontLeftShaft');
      | port_label('input',8, 'FrontRightShaft');
      | port_label('input',9, 'RearDifferential');
      | port_label('input',10, 'RearLeftShaft');
      | port_label('input',11, 'RearRightShaft');
      | port_label('input',12, 'Rear2Differential');
      | port_label('input',13, 'Rear2LeftShaft');
      | port_label('input',14, 'Rear2RightShaft');
      | port_label('input',15, 'Rear3Differential');
      | port_label('input',16, 'Rear3LeftShaft');
      | port_label('input',17, 'Rear3RightShaft');
      | port_label('input',18, 'TotalRatio[-]');
      | port_label('output',1, 'DrivetrainPhysics');
  FrontDifferentialOutput : Subsystem
  FrontLeftShaftOutput : Subsystem
  FrontRightShaftOutput : Subsystem
  Memory : Memory  InheritSampleTime=on
  Memory1 : Memory  InheritSampleTime=on
  Rear2DifferentialOutput : Subsystem
  Rear2LeftShaftOutput : Subsystem
  Rear2RightShaftOutput : Subsystem
  Rear3DifferentialOutput : Subsystem
  Rear3LeftShaftOutput : Subsystem
  Rear3RightShaftOutput : Subsystem
  RearDifferentialOutput : Subsystem
  RearLeftShaftOutput : Subsystem
  RearRightShaftOutput : Subsystem
  Sum : Sum  Inputs=+
  TransferCaseOutput : Subsystem
  TransmissionOutput : Subsystem
  DrivetrainPhysics : Outport  VectorParamsAs1DForOutWhenUnconnected=off
  wires:
  Memory1/1 -> DrivetrainPhysicsOutput/18(TotalRatio[-]___UNIQUE_1)
  Sum/1 -> Memory1/1
  Memory/1 -> DrivetrainPhysicsOutput/1(EngSpd[rad/s]___UNIQUE_1)
  Demux5/1 -> Memory/1
  TransferCaseOutput/1(TransferCase) -> DrivetrainPhysicsOutput/5(TransferCase___UNIQUE_1)
  Demux8/1 -> TransferCaseOutput/1(In2)
  Demux3/2 -> Rear2RightShaftOutput/1(In1)
  Demux3/1 -> Rear2LeftShaftOutput/1(In1)
  Demux1/2 -> RearRightShaftOutput/1(In1)
  Demux1/1 -> RearLeftShaftOutput/1(In1)
  Demux2/2 -> FrontRightShaftOutput/1(In1)
  Demux2/1 -> FrontLeftShaftOutput/1(In1)
  Rear3RightShaftOutput/1(Rear3RightShaft) -> DrivetrainPhysicsOutput/17(Rear3RightShaft___UNIQUE_1)
  Rear3LeftShaftOutput/1(Rear3LeftShaft) -> DrivetrainPhysicsOutput/16(Rear3LeftShaft___UNIQUE_1)
  Rear3DifferentialOutput/1(Rear3Differential) -> DrivetrainPhysicsOutput/15(Rear3Differential___UNIQUE_1)
  Rear2RightShaftOutput/1(Rear2RightShaft) -> DrivetrainPhysicsOutput/14(Rear2RightShaft___UNIQUE_1)
  Rear2LeftShaftOutput/1(Rear2LeftShaft) -> DrivetrainPhysicsOutput/13(Rear2LeftShaft___UNIQUE_1)
  Rear2DifferentialOutput/1(Rear2Differential) -> DrivetrainPhysicsOutput/12(Rear2Differential___UNIQUE_1)
  RearRightShaftOutput/1(RearRightShaft) -> DrivetrainPhysicsOutput/11(RearRightShaft___UNIQUE_1)
  RearLeftShaftOutput/1(RearLeftShaft) -> DrivetrainPhysicsOutput/10(RearLeftShaft___UNIQUE_1)
  RearDifferentialOutput/1(RearDifferential) -> DrivetrainPhysicsOutput/9(RearDifferential___UNIQUE_1)
  FrontRightShaftOutput/1(FrontRightShaft) -> DrivetrainPhysicsOutput/8(FrontRightShaft___UNIQUE_1)
  FrontLeftShaftOutput/1(FrontLeftShaft) -> DrivetrainPhysicsOutput/7(FrontLeftShaft___UNIQUE_1)
  FrontDifferentialOutput/1(FrontDifferential) -> DrivetrainPhysicsOutput/6(FrontDifferential___UNIQUE_1)
  TransmissionOutput/1(Transmission) -> DrivetrainPhysicsOutput/4(Transmission___UNIQUE_1)
  ClutchOutput/1(Clutch) -> DrivetrainPhysicsOutput/3(Clutch___UNIQUE_1)
  DrivetrainPhysicsOutput/1(DrivetrainPhysics___UNIQUE_1) -> DrivetrainPhysics/1
  DrivetrainStates/1 -> Demux7/1
  ShaftStates/1 -> Demux/1
  EngStates/1 -> Demux5/1
  Demux5/2 -> DrivetrainPhysicsOutput/2(EngAcc[rad/s**2]___UNIQUE_1)
  Demux/1 -> Demux2/1
  Demux/2 -> Demux1/1
  Demux/3 -> Demux3/1
  Demux/4 -> Demux6/1
  Demux6/1 -> Rear3LeftShaftOutput/1(In1)
  Demux6/2 -> Rear3RightShaftOutput/1(In1)
  Demux7/1 -> ClutchOutput/1(ClutchStates)
  Demux7/2 -> TransmissionOutput/1(TransmissionStates)
  Demux7/4 -> Sum/1
  Demux8/2 -> FrontDifferentialOutput/1(In2)
  Demux8/3 -> RearDifferentialOutput/1(In2)
  Demux8/4 -> Rear2DifferentialOutput/1(In2)
  Demux8/5 -> Rear3DifferentialOutput/1(In2)
  Demux7/3 -> Demux8/1

== system PassengerCar/Vehicle/Drivetrain/DrivetrainPhysics/DynaComponentInfo ==

== system PassengerCar/Vehicle/Engine/EngineControlUnit/DynaComponentInfo ==
